simulink model "massestimate0x2830x29_other"  (R2023b)
settings: Solver=VariableStepAuto  StartTime=T_start  StopTime=T_stop  FixedStep=T_step  RelTol=1e-3
values from neighbouring files (symbols this model uses):
  BatteryEdensIcecube = 134.4    [Parametersettingscript.m]
  BatteryEdensity1 = 150    [Parametersettingscript.m]
  BatteryEdensity2 = 200    [Parametersettingscript.m]
  BatteryEdensity3 = 400    [Parametersettingscript.m]
  Battmassfrac = 0.2    [Parametersettingscript.m]
  fwdorbwd = ones(arraylength,1)    [Parametersettingscript.m]    (also in Velocityprofiler_test.m)
  lengths = Routesegment(:,3)    [Parametersettingscript.m]    (also in Velocityprofiler_test.m)
  Mass = 800    [Parametersettingscript.m]
  roadcurvatures = zeros(arraylength,1)    [Parametersettingscript.m]    (also in Velocityprofiler_test.m)
  V_end = 6    [Parametersettingscript.m]    (also in Velocityprofiler_test.m = 1)
  V_start = 0    [Parametersettingscript.m]    (also in Velocityprofiler_test.m = 30)
libraries: autolibshared x5, matrix_library x2, drivinglib x1
settings Model: Creator=cas  LastModifiedBy=Jords

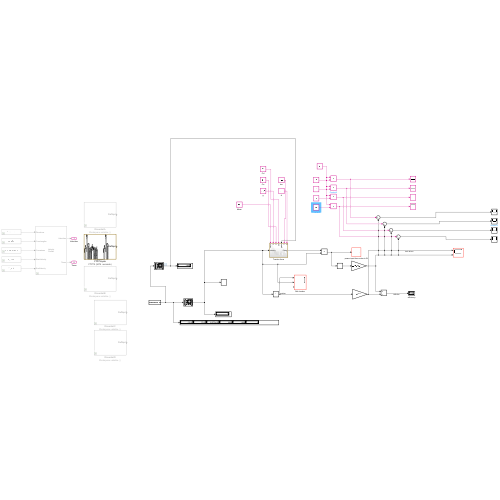
[thumbnail: Simulink's stored preview of the top-level diagram]
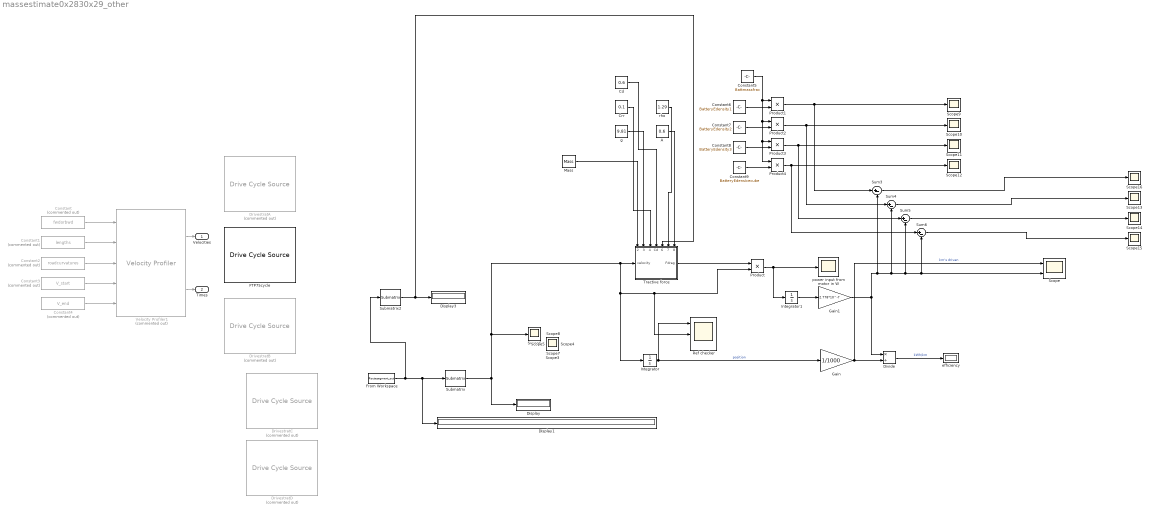
== system massestimate0x2830x29_other ==
  A : Constant  Value=0.6
  Cd : Constant  Value=0.6
  Constant : Constant  Commented=on  Value=fwdorbwd
  Constant1 : Constant  Commented=on  Value=lengths
  Constant2 : Constant  Commented=on  Value=roadcurvatures
  Constant3 : Constant  Commented=on  Value=V_start
  Constant4 : Constant  Commented=on  Value=V_end
  Constant5 : Constant  Value=Battmassfrac
  Constant6 : Constant  Value=BatteryEdensity1
  Constant7 : Constant  Value=BatteryEdensity2
  Constant8 : Constant  Value=BatteryEdensity3
  Constant9 : Constant  Value=BatteryEdensIcecube
  Crr : Constant  Value=0.1
  Display : Display
  Display1 : Display
  Display3 : Display
  Divide : Product  Inputs=*/
  DrivestratA : autolibshared/Drive Cycle Source  Commented=on  cycleVar=Workspace variable  wsVar=DrivestratA  fileVar=cycleFTP75.mat  tfinal=""  cycleRepeat=off  outAccPort=off  outGearPort=off  gearList=No gear data  t_wot1=5  xdot_woto=0  xdot_wot1=5  t_wot2=95  xdot_wot2=0  t_wotend=100  srcUnit=m/s  outUnit=m/s  srcAccUnit=m/s/s  outAccUnit=m/s^2  dt=T_step  aMode=1  faultOption=off  velBnd=2  velBndUnit=mph  inUnit=m/s  timeBnd=1  failOption=off  stopSim=off  maxFaultCnt=10  maxFaultTime=2  maxTotFaultTime=15  traceOption=off  dtTrace=1  traceWindow=10  lastDCname=Custom Data Set  lastOutUnit=mph  lastDT=T_step  lastTB=1  lastSB=2  forceCalcBound=off
  DrivestratB : autolibshared/Drive Cycle Source  Commented=on  cycleVar=Workspace variable  wsVar=DrivestratA  fileVar=cycleFTP75.mat  tfinal=""  cycleRepeat=off  outAccPort=off  outGearPort=off  gearList=No gear data  t_wot1=5  xdot_woto=0  xdot_wot1=5  t_wot2=95  xdot_wot2=0  t_wotend=100  srcUnit=m/s  outUnit=m/s  srcAccUnit=m/s/s  outAccUnit=m/s^2  dt=T_step  aMode=1  faultOption=off  velBnd=2  velBndUnit=mph  inUnit=m/s  timeBnd=1  failOption=off  stopSim=off  maxFaultCnt=10  maxFaultTime=2  maxTotFaultTime=15  traceOption=off  dtTrace=1  traceWindow=10  lastDCname=Custom Data Set  lastOutUnit=mph  lastDT=T_step  lastTB=1  lastSB=2  forceCalcBound=off
  DrivestratC : autolibshared/Drive Cycle Source  Commented=on  cycleVar=Workspace variable  wsVar=DrivestratA  fileVar=cycleFTP75.mat  tfinal=""  cycleRepeat=off  outAccPort=off  outGearPort=off  gearList=No gear data  t_wot1=5  xdot_woto=0  xdot_wot1=5  t_wot2=95  xdot_wot2=0  t_wotend=100  srcUnit=m/s  outUnit=m/s  srcAccUnit=m/s/s  outAccUnit=m/s^2  dt=T_step  aMode=1  faultOption=off  velBnd=2  velBndUnit=mph  inUnit=m/s  timeBnd=1  failOption=off  stopSim=off  maxFaultCnt=10  maxFaultTime=2  maxTotFaultTime=15  traceOption=off  dtTrace=1  traceWindow=10  lastDCname=Custom Data Set  lastOutUnit=mph  lastDT=T_step  lastTB=1  lastSB=2  forceCalcBound=off
  DrivestratD : autolibshared/Drive Cycle Source  Commented=on  cycleVar=Workspace variable  wsVar=DrivestratA  fileVar=cycleFTP75.mat  tfinal=""  cycleRepeat=off  outAccPort=off  outGearPort=off  gearList=No gear data  t_wot1=5  xdot_woto=0  xdot_wot1=5  t_wot2=95  xdot_wot2=0  t_wotend=100  srcUnit=m/s  outUnit=m/s  srcAccUnit=m/s/s  outAccUnit=m/s^2  dt=T_step  aMode=1  faultOption=off  velBnd=2  velBndUnit=mph  inUnit=m/s  timeBnd=1  failOption=off  stopSim=off  maxFaultCnt=10  maxFaultTime=2  maxTotFaultTime=15  traceOption=off  dtTrace=1  traceWindow=10  lastDCname=Custom Data Set  lastOutUnit=mph  lastDT=T_step  lastTB=1  lastSB=2  forceCalcBound=off
  FTP75cycle : autolibshared/Drive Cycle Source  cycleVar=FTP75  fileVar=cycleFTP75.mat  tfinal="2474  seconds"  cycleRepeat=off  outAccPort=off  outGearPort=off  gearList=No gear data  t_wot1=5  xdot_woto=0  xdot_wot1=5  t_wot2=95  xdot_wot2=0  t_wotend=100  srcUnit=m/s  outUnit=m/s  srcAccUnit=m/s/s  outAccUnit=m/s^2  dt=0  aMode=1  faultOption=off  velBnd=2  velBndUnit=mph  inUnit=m/s  timeBnd=1  failOption=off  stopSim=off  maxFaultCnt=10  maxFaultTime=2  maxTotFaultTime=15  traceOption=off  dtTrace=1  traceWindow=10  lastDCname=FTP75  lastOutUnit=mph  lastDT=0  lastTB=1  lastSB=2  forceCalcBound=off
  From Workspace : FromWorkspace  VariableName=Routesegment_out  OutDataTypeStr=double
  Gain : Gain  Gain=1/1000
  Gain1 : Gain  Gain=2.778*10^-7
  Integrator : Integrator
  Integrator1 : Integrator
  Mass : Constant  Value=Mass
  Product{,1..4} (5 alike) : Product
  Ref checker : Scope  NumInputPorts=3
  Scope : Scope  NumInputPorts=2
  Scope{1..16} (16 alike) : Scope
  Submatrix : matrix_library/Submatrix  RowSpan=One row  RowStartMode=Last  RowStartIndex=1  RowEndMode=Last  RowEndIndex=1  ColSpan=All columns  ColStartMode=First  ColStartIndex=5  ColEndMode=Last  ColEndIndex=1
  Submatrix2 : matrix_library/Submatrix  RowSpan=One row  RowStartMode=Offset from last  RowStartIndex=1  RowEndMode=Last  RowEndIndex=1  ColSpan=All columns  ColStartMode=First  ColStartIndex=5  ColEndMode=Last  ColEndIndex=1
  Sum{3..6} (4 alike) : Sum  Inputs=|+-
  Tractive force : Subsystem
      settings: PortSchema="{\"entries\":[{\"content\":{\"sides\":[{\"content\":{\"connectorIds\":[\"In1\"]},\"type\":\"ConnectorPlacement.EquallySpacedRectSide\",\"uuid\":\"1dc941f5-3e74-4cbf-a52e-ea3cab36909e\"},{\"content\":{\"connectorIds\":[\"Out1\"],\"side\":\"RIGHT\"},\"type\":\"ConnectorPlacement.EquallySpacedRectSide\",\"uuid\":\"6f8e9dcb-b594-405f-a2b1-c41d344efafb\"},{\"content\":{\"connectorIds\":[\"In2\",\"In3\",\"In4\",\"In5\",\"In6\",\"In7\",\"In8\"],\"side\":\"TOP\"},\"type\":\"ConnectorPlacement.EquallySpacedRectSide\",\"uuid\":\"1ae95007-d3a7-4d64-89c5-5ad33b1ab93d\"}]},\"type\":\"ConnectorPlacement.EquallySpacedConnector\",\"uuid\":\"adcee74b-2e32-4cf6-bb91-c8e1408d67ea\"}],\"packageUris\":[\"http://schema.mathworks.com/mf0/Connector/R2020b\"],\"version\":\"1.0\"}"
  Velocity Profiler1 : drivinglib/Velocity Profiler  Commented=on  MaxLongitudinalAccel=3  MaxLongitudinalDecel=1  MaxSpeed=maxspeed  MaxLongitudinalJerk=1  MaxLateralAccel=1  ShowOptionalOutport=on  SampleTime=0.1  SimulateUsing=Code generation
  efficiency : Display
      settings: Format=bank
  g : Constant  Value=9.81
  power input from motor in W : Scope
  rho : Constant  Value=1.29
  Velocities : Outport  VectorParamsAs1DForOutWhenUnconnected=off
  Times : Outport  Port=2  VectorParamsAs1DForOutWhenUnconnected=off
  wires:
  Gain/1 -> Scope/1, Divide/2  "km's driven"
  Divide/1 -> efficiency/1  "kWh/km"
  Product/1 -> Integrator1/1, power input from motor in W/1
  Integrator/1 -> Ref checker/1, Gain/1  "position"
  Tractive force/1(Fdrag) -> Product/1
  Gain1/1 -> Divide/1, Sum4/2, Sum5/2, Scope/2, Sum6/2, Sum3/2
  Integrator1/1 -> Gain1/1
  Mass/1 -> Tractive force/2(mass)
  g/1 -> Tractive force/3(In3)
  Crr/1 -> Tractive force/4(In4)
  Cd/1 -> Tractive force/5(Cd)
  rho/1 -> Tractive force/7(In7)
  A/1 -> Tractive force/8(In8)
  Constant2/1 -> Velocity Profiler1/3
  Constant3/1 -> Velocity Profiler1/4
  Constant4/1 -> Velocity Profiler1/5
  Velocity Profiler1/2 -> Times/1
  Velocity Profiler1/1 -> Velocities/1
  Constant/1 -> Velocity Profiler1/1
  Constant1/1 -> Velocity Profiler1/2
  From Workspace/1 -> Submatrix2/1, Submatrix/1, Display1/1
  Submatrix/1 -> Integrator/1, Ref checker/2, Product/2, Tractive force/1(velocity), Scope6/1, Display/1
  Submatrix2/1 -> Tractive force/6(grade), Display3/1
  Constant5/1 -> Product4/1, Product3/1, Product2/1, Product1/1
  Product4/1 -> Sum6/1, Scope12/1
  Product1/1 -> Sum3/1, Scope9/1
  Product2/1 -> Sum4/1, Scope10/1
  Product3/1 -> Sum5/1, Scope11/1
  Constant6/1 -> Product1/2
  Constant9/1 -> Product4/2
  Constant7/1 -> Product2/2
  Constant8/1 -> Product3/2
  Sum4/1 -> Scope13/1
  Sum6/1 -> Scope15/1
  Sum5/1 -> Scope14/1
  Sum3/1 -> Scope16/1

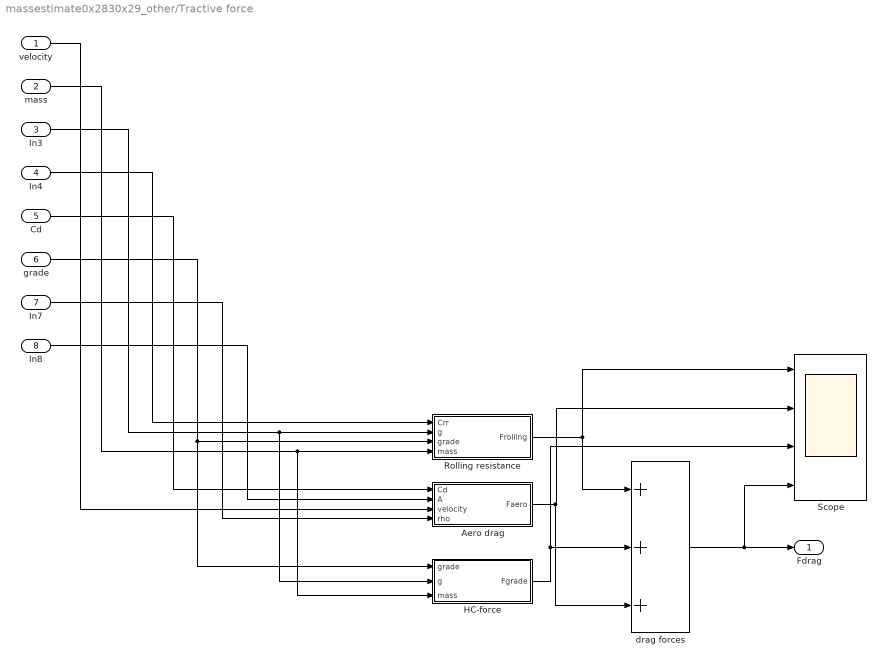
== system massestimate0x2830x29_other/Tractive force ==
  velocity : Inport
  mass : Inport  Port=2
  In3 : Inport  Port=3
  In4 : Inport  Port=4
  Cd : Inport  Port=5
  grade : Inport  Port=6
  In7 : Inport  Port=7
  In8 : Inport  Port=8
  Aero drag : Subsystem
  HC-force : Subsystem
  Rolling resistance : Subsystem
  Scope : Scope  NumInputPorts=4
  drag forces : Sum  Inputs=+++
  Fdrag : Outport
  wires:
  Rolling resistance/1(Frolling) -> drag forces/1, Scope/1
  HC-force/1(Fgrade) -> Scope/3, drag forces/2
  drag forces/1 -> Scope/4, Fdrag/1
  Aero drag/1(Faero) -> drag forces/3, Scope/2
  velocity/1 -> Aero drag/3(velocity)
  mass/1 -> HC-force/3(mass), Rolling resistance/4(mass)
  In3/1 -> HC-force/2(g), Rolling resistance/2(g)
  In4/1 -> Rolling resistance/1(Crr)
  Cd/1 -> Aero drag/1(Cd)
  grade/1 -> HC-force/1(grade), Rolling resistance/3(grade)
  In7/1 -> Aero drag/4(rho)
  In8/1 -> Aero drag/2(A)

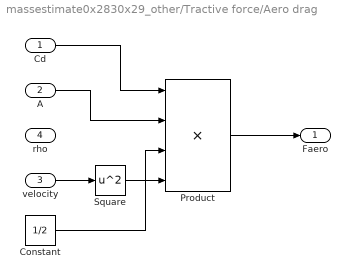
== system massestimate0x2830x29_other/Tractive force/Aero drag ==
  Cd : Inport
  A : Inport  Port=2
  velocity : Inport  Port=3
  rho : Inport  Port=4
  Constant : Constant  Value=1/2
  Product : Product  Inputs=4
  Square : Math  Operator=square
  Faero : Outport
  wires:
  Cd/1 -> Product/1
  velocity/1 -> Square/1
  A/1 -> Product/2
  Square/1 -> Product/4
  Constant/1 -> Product/3
  Product/1 -> Faero/1

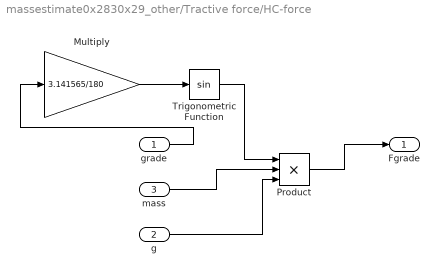
== system massestimate0x2830x29_other/Tractive force/HC-force ==
  grade : Inport
  g : Inport  Port=2
  mass : Inport  Port=3
  Multiply : Gain  Gain=3.141565/180
  Product : Product  Inputs=3
  Trigonometric Function : Trigonometry
  Fgrade : Outport
  wires:
  grade/1 -> Multiply/1
  Multiply/1 -> Trigonometric Function/1
  Trigonometric Function/1 -> Product/1
  mass/1 -> Product/2
  g/1 -> Product/3
  Product/1 -> Fgrade/1

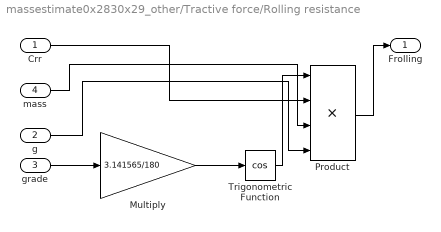
== system massestimate0x2830x29_other/Tractive force/Rolling resistance ==
  Crr : Inport
  g : Inport  Port=2
  grade : Inport  Port=3
  mass : Inport  Port=4
  Multiply : Gain  Gain=3.141565/180
  Product : Product  Inputs=4
  Trigonometric Function : Trigonometry  Operator=cos
  Frolling : Outport
  wires:
  Crr/1 -> Product/2
  mass/1 -> Product/3
  g/1 -> Product/4
  grade/1 -> Multiply/1
  Multiply/1 -> Trigonometric Function/1
  Trigonometric Function/1 -> Product/1
  Product/1 -> Frolling/1
